simulink model "ObsPertContinuoRed"  (R2022b)
settings: Solver=ode45  StartTime=0.0  StopTime=700  RelTol=1e-8  EnableMultiTasking=on
values from neighbouring files (symbols this model uses):
  Lp = Lp    [PrObsPertContinuoRed.m]
  Lr1 = L(2)    [PrObsPertContinuoRed.m]
  Lr2 = L(3)    [PrObsPertContinuoRed.m]
  Ls1 = L(4)    [PrObsPertContinuoRed.m]    (also in TestesEEobsPert.m = L(5))
  Ls2 = L(5)    [PrObsPertContinuoRed.m]    (also in TestesEEobsPert.m = L(6))
settings Model: Creator=adolfobs  LastModifiedBy=adolfo
settings SolverCC: AlgebraicLoopSolver=TrustRegion
settings DataIOCC: LimitDataPoints=on  MaxDataPoints=25000  SaveFormat=Array  SignalLoggingSaveFormat=ModelDataLogs  ReturnWorkspaceOutputs=off
settings OptimizationCC: BlockReduction=off  BooleanDataType=off  InitFltsAndDblsToZero=on  LifeSpan=inf
settings DebuggingCC: SaveWithParameterizedLinksMsg=none  UnderspecifiedInitializationDetection=Classic  MergeDetectMultiDrivingBlocksExec=none  SignalResolutionControl=TryResolveAllWithWarning  MultiTaskDSMMsg=warning  MultiTaskCondExecSysMsg=none  UnconnectedInputMsg=warning  UnconnectedOutputMsg=warning  UnconnectedLineMsg=warning  SFUnexpectedBacktrackingDiag=warning  SFNoUnconditionalDefaultTransitionDiag=warning  SFExecutionAtInitializationDiag=none  SFMachineParentedDataDiag=warning  ArithmeticOperatorsInVariantConditions=warning
settings HardwareCC: ProdBitPerPointer=32  ProdBitPerSizeT=32  ProdBitPerPtrDiffT=32  ProdLargestAtomicFloat=None  ProdIntDivRoundTo=Undefined  ProdEndianess=Unspecified  ProdWordSize=32  ProdHWDeviceType=32-bit Generic  TargetUnknown=on
settings ModelReferenceCC: EnableRefExpFcnMdlSchedulingChecks=on  PropagateSignalLabelsOutOfModel=off
settings SFSimCC: SimUseLocalCustomCode=off  CustomCodeUndefinedFunction=UseInterfaceOnly
settings RTWCC: RTWUseLocalCustomCode=off
settings CodeAppCC: StateflowObjectComments=on
settings GRTTargetCC: TargetFcnLib=ansi_tfl_tmw.mat  TargetLangStandard=C89/C90 (ANSI)  CombineOutputUpdateFcns=off  GRTInterface=on
settings ConfigComp: CovMetricSettings=dw  CovSaveCumulativeToWorkspaceVar=on  CovSaveSingleToWorkspaceVar=on  CovExternalEMLEnable=off

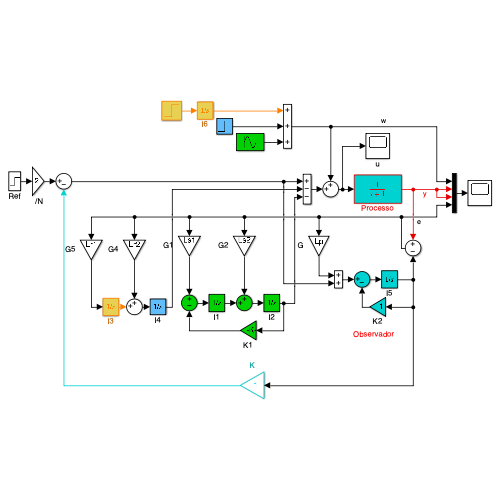
[thumbnail: Simulink's stored preview of the top-level diagram]
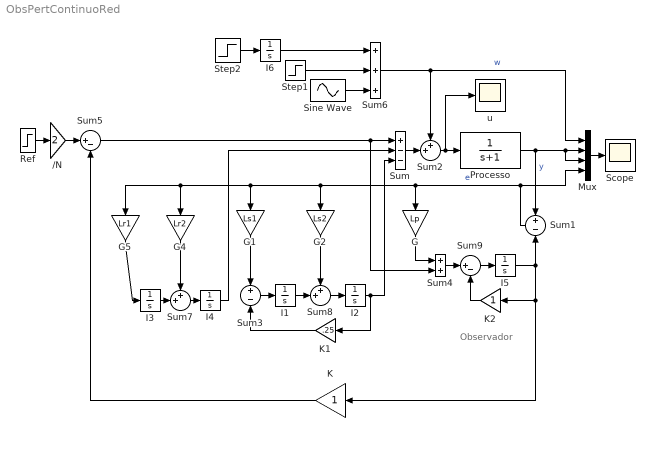
== system ObsPertContinuoRed ==
  note: Observador
  " /N" : Gain  Gain=2  SaturateOnIntegerOverflow=on  OutDataTypeStr=Inherit: Same as input  ParamDataTypeStr=Inherit: Same as input
  G : Gain  Gain=Lp  SaturateOnIntegerOverflow=on  OutDataTypeStr=Inherit: Same as input  ParamDataTypeStr=Inherit: Same as input
  G1 : Gain  Gain=Ls1  SaturateOnIntegerOverflow=on  OutDataTypeStr=Inherit: Same as input  ParamDataTypeStr=Inherit: Same as input
  G2 : Gain  Gain=Ls2  SaturateOnIntegerOverflow=on  OutDataTypeStr=Inherit: Same as input  ParamDataTypeStr=Inherit: Same as input
  G4 : Gain  Gain=Lr2  SaturateOnIntegerOverflow=on  OutDataTypeStr=Inherit: Same as input  ParamDataTypeStr=Inherit: Same as input
  G5 : Gain  Gain=Lr1  SaturateOnIntegerOverflow=on  OutDataTypeStr=Inherit: Same as input  ParamDataTypeStr=Inherit: Same as input
  I{1..6} (6 alike) : Integrator
  K : Gain  SaturateOnIntegerOverflow=on  OutDataTypeStr=Inherit: Same as input  ParamDataTypeStr=Inherit: Same as input
  K1 : Gain  Gain=.25  SaturateOnIntegerOverflow=on  OutDataTypeStr=Inherit: Same as input  ParamDataTypeStr=Inherit: Same as input
  K2 : Gain  SaturateOnIntegerOverflow=on  OutDataTypeStr=Inherit: Same as input  ParamDataTypeStr=Inherit: Same as input
  Mux : Mux
  Processo : TransferFcn  Denominator=[1 1]
  Ref : Step  Time=100  SampleTime=0
  Scope : Scope
  Sine Wave : Sin  Amplitude=.3  Frequency=.5
  Step1 : Step  Time=140  After=.2
  Step2 : Step  Time=400  After=.01  SampleTime=0
  Sum : Sum  Inputs=+--  InputSameDT=on  SaturateOnIntegerOverflow=on  OutDataTypeStr=Inherit: Same as first input
  Sum1 : Sum  Inputs=+-  InputSameDT=on  SaturateOnIntegerOverflow=on  OutDataTypeStr=Inherit: Same as first input
  Sum2 : Sum  Inputs=++|  InputSameDT=on  SaturateOnIntegerOverflow=on  OutDataTypeStr=Inherit: Same as first input
  Sum3 : Sum  Inputs=+|-  InputSameDT=on  SaturateOnIntegerOverflow=on  OutDataTypeStr=Inherit: Same as first input
  Sum4 : Sum  InputSameDT=on  SaturateOnIntegerOverflow=on  OutDataTypeStr=Inherit: Same as first input
  Sum5 : Sum  Inputs=|+-  InputSameDT=on  SaturateOnIntegerOverflow=on  OutDataTypeStr=Inherit: Same as first input
  Sum6 : Sum  Inputs=+++  InputSameDT=on  SaturateOnIntegerOverflow=on  OutDataTypeStr=Inherit: Same as first input
  Sum7 : Sum  Inputs=++|  InputSameDT=on  SaturateOnIntegerOverflow=on  OutDataTypeStr=Inherit: Same as first input
  Sum8 : Sum  Inputs=++|  InputSameDT=on  SaturateOnIntegerOverflow=on  OutDataTypeStr=Inherit: Same as first input
  Sum9 : Sum  Inputs=|+-  InputSameDT=on  SaturateOnIntegerOverflow=on  OutDataTypeStr=Inherit: Same as first input
  u : Scope
  wires:
  Sum2/1 -> u/1, Processo/1
  Sum/1 -> Sum2/2
  Mux/1 -> Scope/1
  Sum1/1 -> Mux/4, G2/1, G5/1, G4/1, G1/1, G/1  "e"
  Sum3/1 -> I1/1
  I2/1 -> K1/1, Sum/3
  I5/1 -> Sum1/2, K2/1, K/1
  Sum4/1 -> Sum9/1
  G/1 -> Sum4/1
  G1/1 -> Sum3/1
  K/1 -> Sum5/2
  Processo/1 -> Sum1/1, Mux/2, Mux/3  "y"
  Ref/1 -> " /N"/1
  " /N"/1 -> Sum5/1
  Sum6/1 -> Mux/1, Sum2/1  "w"
  G5/1 -> I3/1
  I3/1 -> Sum7/2
  Sine Wave/1 -> Sum6/3
  Step1/1 -> Sum6/2
  Step2/1 -> I6/1
  I6/1 -> Sum6/1
  K1/1 -> Sum3/2
  Sum5/1 -> Sum/1, Sum4/2
  G4/1 -> Sum7/1
  Sum7/1 -> I4/1
  G2/1 -> Sum8/1
  Sum8/1 -> I2/1
  I1/1 -> Sum8/2
  I4/1 -> Sum/2
  K2/1 -> Sum9/2
  Sum9/1 -> I5/1
